simulink model "koord_razv"  (R2022b)
settings: Solver=VariableStepAuto  StartTime=0.0  StopTime=3  RelTol=1e-3
values from neighbouring files (symbols this model uses):
  g_del_V = 0.051    [NA_ZACHET.m]    (also in koord_razv.m)
  k_omx = x(1)    [koord_razv.m]
  k_psi_e = x(3)    [koord_razv.m]
  k_sigm = x(2)    [koord_razv.m]
  kzi_pr = 0.707    [NA_ZACHET.m]    (also in koord_razv.m)
  M_x_omx = -1    [NA_ZACHET.m]    (also in koord_razv.m)
  M_x_sigme = -7    [NA_ZACHET.m]    (also in koord_razv.m)
  om_pr = 20    [NA_ZACHET.m]    (also in koord_razv.m)
libraries: checkpacklib x1
settings Model: Creator=79251  LastModifiedBy=79251

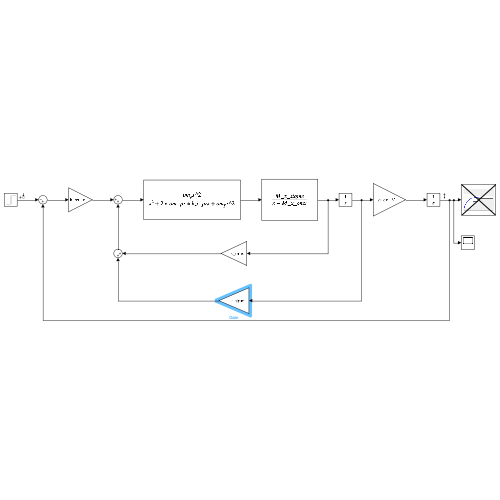
[thumbnail: Simulink's stored preview of the top-level diagram]
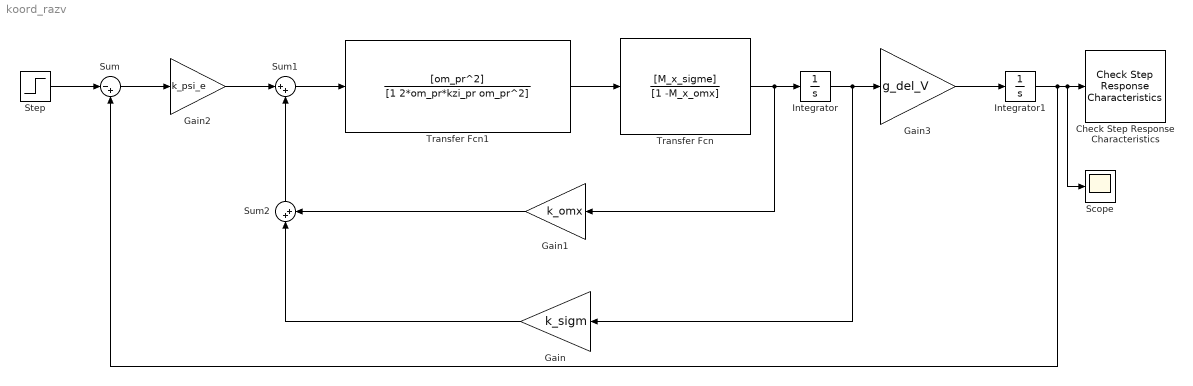
== system koord_razv ==
  Check Step Response Characteristics : checkpacklib/Check Step Response  Characteristics  InstantiateOnLoad=on  enabled=off  stopWhenAssertionFail=off  export=off  ViewDlgPos=[]  OpenViewOnLoad=off  LaunchViewOnOpen=off  TimeUnits=seconds  EnableStepResponseBound=on  InitialValue=0  FinalValue=1  StepTime=0  RiseTime=0.8  PercentRise=50  SettlingTime=1  PercentSettling=5  PercentOvershoot=5  PercentUndershoot=5
      settings: LibrarySourceBlock=|
      | sdolib/Model Verification/Check Step Response
      | Characteristics
  Gain : Gain  Gain=k_sigm
  Gain1 : Gain  Gain=k_omx
  Gain2 : Gain  Gain=k_psi_e
  Gain3 : Gain  Gain=g_del_V
  Integrator : Integrator
  Integrator1 : Integrator
  Scope : Scope
  Step : Step  Time=0  SampleTime=0
  Sum : Sum  Inputs=|-+
  Sum1 : Sum  Inputs=|++
  Sum2 : Sum  Inputs=|++
  Transfer Fcn : TransferFcn  Numerator=[M_x_sigme]  Denominator=[1 -M_x_omx]
  Transfer Fcn1 : TransferFcn  Numerator=[om_pr^2]  Denominator=[1 2*om_pr*kzi_pr om_pr^2]
  wires:
  Gain3/1 -> Integrator1/1
  Transfer Fcn/1 -> Gain1/1, Integrator/1
  Integrator/1 -> Gain/1, Gain3/1
  Integrator1/1 -> Sum/2, Scope/1, Check Step Response Characteristics/1
  Gain1/1 -> Sum2/2
  Gain/1 -> Sum2/1
  Sum2/1 -> Sum1/2
  Sum1/1 -> Transfer Fcn1/1
  Gain2/1 -> Sum1/1
  Sum/1 -> Gain2/1
  Step/1 -> Sum/1
  Transfer Fcn1/1 -> Transfer Fcn/1
